simulink model "SimpleStateFlow"  (R2024a)
settings: Solver=FixedStepDiscrete  StartTime=0.0  StopTime=inf  FixedStep=1  RelTol=1e-3
settings Model: Creator=sscsh  LastModifiedBy=sscsh
settings OptimizationCC: DefaultParameterBehavior=Inlined  UseDivisionForNetSlopeComputation=on  GainParamInheritBuiltInType=on  UseFloatMulNetSlope=on  InlineInvariantSignals=on  PassReuseOutputArgsAs=Individual arguments  ZeroExternalMemoryAtStartup=off  ZeroInternalMemoryAtStartup=off  NoFixptDivByZeroProtection=on  EfficientFloat2IntCast=on  LifeSpan=1  OptimizeBlockOrder=speed  DifferentSizesBufferReuse=on  EfficientTunableParamExpr=on
settings DebuggingCC: ParameterTunabilityLossMsg=error
settings HardwareCC: ProdBitPerPointer=32  ProdBitPerSizeT=32  ProdBitPerPtrDiffT=32  ProdLargestAtomicInteger=Long  ProdLargestAtomicFloat=Double  ProdWordSize=32  ProdLongLongMode=on  ProdHWDeviceType=Texas Instruments->Stellaris Cortex-M3
settings SFSimCC: MATLABDynamicMemAlloc=off
settings RTWCC: Description=Embedded Coder  SystemTargetFile=ert.tlc  TemplateMakefile=ert_default_tmf
settings CodeAppCC: ForceParamTrailComments=on  IgnoreCustomStorageClasses=off  OperatorAnnotations=on  SimulinkDataObjDesc=on  SFDataObjDesc=on  CustomSymbolStrGlobalVar=rt$N$M  CustomSymbolStrType=$N$M  CustomSymbolStrFcn=$N$M$F  CustomSymbolStrMacro=$N$M  InsertBlockDesc=on
settings ERTTargetCC: TargetLangStandard=C99 (ISO)  GenerateSampleERTMain=on  IncludeMdlTerminateFcn=off  CombineSignalStateStructs=on  SupportAbsoluteTime=off  CodeInterfacePackaging=Reusable function  SupportComplex=off  SupportNonInlinedSFcns=on  InlinedParameterPlacement=NonHierarchical  ERTCustomFileTemplate=example_file_process.tlc  ERTFilePackagingFormat=CompactWithDataFile

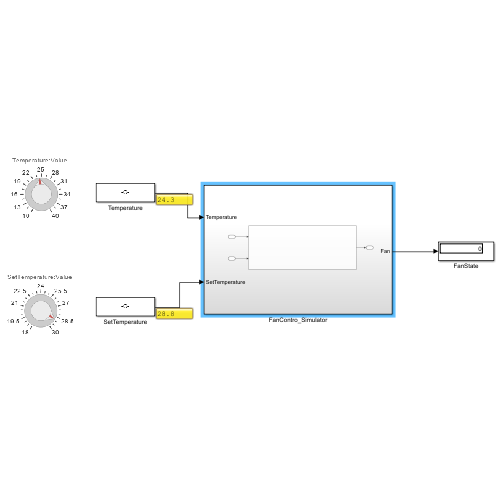
[thumbnail: Simulink's stored preview of the top-level diagram]
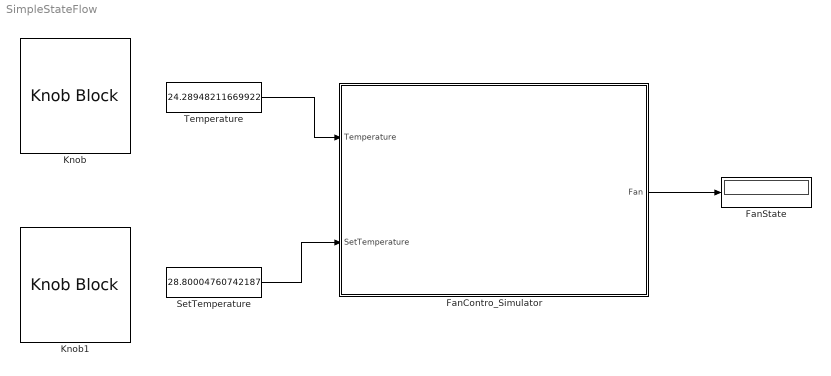
== system SimpleStateFlow ==
  FanContro_Simulator : Subsystem
  FanState : Display
  Knob : KnobBlock  ScaleMin=10  ScaleMax=40
  Knob1 : KnobBlock  ScaleMin=18  ScaleMax=30
  SetTemperature : Constant  Value=28.80004760742187
  Temperature : Constant  Value=24.28948211669922
  wires:
  SetTemperature/1 -> FanContro_Simulator/2(SetTemperature)
  Temperature/1 -> FanContro_Simulator/1(Temperature)
  FanContro_Simulator/1(Fan) -> FanState/1

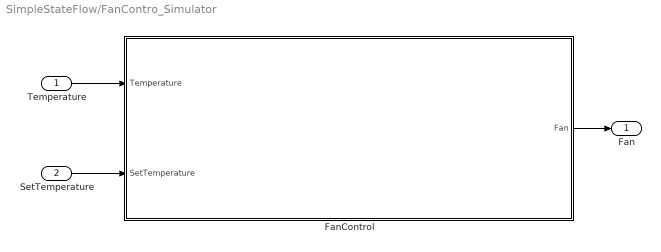
== system SimpleStateFlow/FanContro_Simulator ==
  Temperature : Inport  OutDataTypeStr=double  Unit=°C
  SetTemperature : Inport  Port=2  OutDataTypeStr=double  Unit=°C
  FanControl : Subsystem
  Fan : Outport  OutMin=0  OutMax=1  OutDataTypeStr=int8
  wires:
  Temperature/1 -> FanControl/1(Temperature)
  SetTemperature/1 -> FanControl/2(SetTemperature)
  FanControl/1(Fan) -> Fan/1

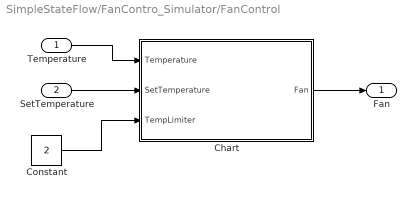
== system SimpleStateFlow/FanContro_Simulator/FanControl ==
  Temperature : Inport
  SetTemperature : Inport  Port=2
  Chart : Stateflow chart  TreatAsAtomicUnit=on
  Constant : Constant  Value=2
  Fan : Outport
  wires:
  Chart/1(Fan) -> Fan/1
  SetTemperature/1 -> Chart/2(SetTemperature)
  Temperature/1 -> Chart/1(Temperature)
  Constant/1 -> Chart/3(TempLimiter)

== stateflow chart SimpleStateFlow/FanContro_Simulator/FanControl/Chart ==
  state FanOn
    entry:
    Fan = 1;
    during:
    Fan = 1;
    exit:
    Fan = 0;;
  state OnStart
    entry:
    Fan = 0;
    during:
    Fan = 0;
    exit:
    Fan = 1;
  (default) -> OnStart
  OnStart -> FanOn : [Temperature > SetTemperature]
  FanOn -> OnStart [order 2] : [ (SetTemperature - TempLimiter) > Temperature ]
  FanOn -> OnStart [order 1] : [Temperature < (SetTemperature - TempLimiter)]
  data: Temperature input; Fan output int8; SetTemperature input; TempLimiter input
